simulink model "velocityMode"  (R2022a)
settings: Solver=FixedStepAuto  StartTime=0.0  StopTime=simTime  FixedStep=samplingTime  RelTol=1e-3
values from neighbouring files (symbols this model uses):
  coulombTorqueNegative = theta(4)/theta(2)    [LeastSquare.m]    (also in leastSquare.m; velRide.m = resultFitNeg(2))
  coulombTorquePositive = theta(3)/theta(2)    [LeastSquare.m]    (also in leastSquare.m; velRide.m = resultFitPos(2))
  inertia = 1/K_w    [LeastSquare.m]    (also in leastSquare.m)
  viscousDamping = -inertia*p_w    [LeastSquare.m]    (also in leastSquare.m; velRide.m = (viscousDampingPos+viscousDampingNeg)/2; velocityRide.m = (viscousDampingPos+viscousDampingNeg)/2)
libraries: slpidlib x1
settings Model: Creator=kose  LastModifiedBy=kose
settings DataIOCC: SaveFormat=Array

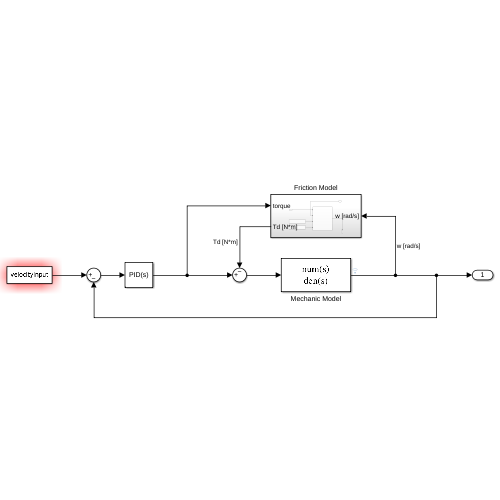
[thumbnail: Simulink's stored preview of the top-level diagram]
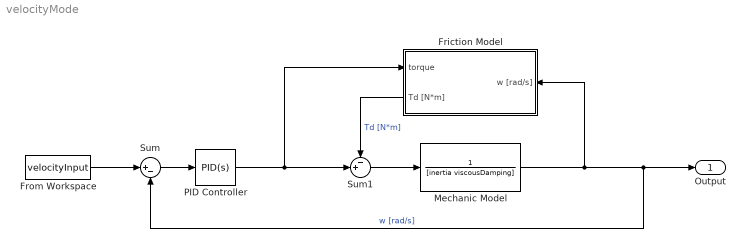
== system velocityMode ==
  Friction Model : Subsystem
      settings: PortSchema="{\"entries\":[{\"content\":{\"sides\":[{\"content\":{\"connectorIds\":[\"In1\"]},\"type\":\"ConnectorPlacement.EquallySpacedRectSide\",\"uuid\":\"8173ecdf-76e4-4809-8dcd-ec0655641a82\"},{\"content\":{\"connectorIds\":[\"In2\",\"Out1\"],\"side\":\"RIGHT\"},\"type\":\"ConnectorPlacement.EquallySpacedRectSide\",\"uuid\":\"02bfb555-c54c-45db-8ee8-f3cb4a7ead24\"},{\"content\":{\"connectorIds\":[],\"side\":\"TOP\"},\"type\":\"ConnectorPlacement.EquallySpacedRectSide\",\"uuid\":\"776da3c7-b053-4a98-8e1b-c60377d5559b\"}]},\"type\":\"ConnectorPlacement.EquallySpacedConnector\",\"uuid\":\"773d656e-d403-490b-8d7a-ce1c081af26d\"}],\"packageUris\":[\"http://schema.mathworks.com/mf0/Connector/R2020b\"],\"version\":\"1.0\"}"
  From Workspace : FromWorkspace  VariableName=velocityInput
  Mechanic Model : TransferFcn  Denominator=[inertia viscousDamping]
  PID Controller : slpidlib/PID Controller  Controller=PID  Form=Parallel  TimeDomain=Continuous-time  UseExternalTs=off  SampleTime=-1  IntegratorMethod=Forward Euler  FilterMethod=Forward Euler  ControllerParametersSource=internal  P=1  I=1  UseKiTs=off  D=0  N=100  UseFilter=on  TunerSelectOption=Transfer Function Based (PID Tuner App)  InitialConditionSource=internal  InitialConditionForIntegrator=0  InitialConditionForFilter=0  DifferentiatorICPrevScaledInput=0  ExternalReset=none  TrackingMode=off  Kt=1  LimitOutput=off  SatLimitsSource=internal  UpperSaturationLimit=inf  LowerSaturationLimit=-inf  LinearizeAsGain=on  AntiWindupMode=none  Kb=1  POutMin=[]  POutMax=[]  IOutMin=[]  IOutMax=[]  DOutMin=[]  DOutMax=[]  NOutMin=[]  NOutMax=[]  SumOutMin=[]  SumOutMax=[]  SaturationOutMin=[]  SaturationOutMax=[]  PParamMin=[]  PParamMax=[]  IParamMin=[]  IParamMax=[]  DParamMin=[]  DParamMax=[]  NParamMin=[]  NParamMax=[]  KbParamMin=[]  KbParamMax=[]  KtParamMin=[]  KtParamMax=[]  KbOutMin=[]  KbOutMax=[]  KtOutMin=[]  KtOutMax=[]  IntegratorOutMin=[]  IntegratorOutMax=[]  FilterOutMin=[]  FilterOutMax=[]  SumI1OutMin=[]  SumI1OutMax=[]  SumI2OutMin=[]  SumI2OutMax=[]  SumI3OutMin=[]  SumI3OutMax=[]  SumI4OutMin=[]  SumI4OutMax=[]  SumDOutMin=[]  SumDOutMax=[]  DifferentiatorOutMin=[]  DifferentiatorOutMax=[]  FilterDiffOutCoefMin=[]  FilterDiffOutCoefMax=[]  ReciprocalOutMin=[]  ReciprocalOutMax=[]  SumDenOutMin=[]  SumDenOutMax=[]  SumNumOutMin=[]  SumNumOutMax=[]  DivideOutMin=[]  DivideOutMax=[]  UdiffTsProdOutMin=[]  UdiffTsProdOutMax=[]  NTsProdOutMin=[]  NTsProdOutMax=[]  UintegralTsProdOutMin=[]  UintegralTsProdOutMax=[]  UngainTsProdOutMin=[]  UngainTsProdOutMax=[]  IntegratorContinuousStateAttributes=''  IntegratorStateMustResolveToSignalObject=off  IntegratorRTWStateStorageClass=Auto  FilterContinuousStateAttributes=''  FilterStateMustResolveToSignalObject=off  FilterRTWStateStorageClass=Auto  ParallelPVariant=InternalParameters  IdealPVariant=Disabled  IVariant=InternalParameters  DVariant=InternalParameters  IntegratorVariant=Continuous  SatVariant=Disabled  AWVariant=Passthrough  PCopyVariant=Disabled  TRVariant=Disabled  FdbkBlocksVariant=Forward  IdealPFdbkVariant=Disabled  SatFdbkVariant=Disabled  DerivativeFilterVariant=ContFilter  NVariant=InternalParameters  NCopyVariant=Disabled  FilterICVariant=InternalICsFilter  IntegratorICVariant=InternalICs  ExternalResetVariant=Disabled  TRSumVariant=Passthrough  SumFdbkVariant=Disabled  SumVariant=Sum_PID  TsampFilterVariant=InternalTs  TsampNgainVariant=Passthrough  TsampIntegralVariant=Passthrough  ExternalSaturationOutDataTypeStr=Inherit: Same as second input  aMode=0
  Sum : Sum  Inputs=|+-
  Sum1 : Sum  Inputs=-+|
  Output : Outport
  wires:
  Mechanic Model/1 -> Friction Model/1(w [rad/s]), Output/1, Sum/2  "w [rad/s]"
  Sum1/1 -> Mechanic Model/1
  Friction Model/1(Td [N*m]) -> Sum1/1  "Td [N*m]"
  PID Controller/1 -> Friction Model/2(torque), Sum1/2
  Sum/1 -> PID Controller/1
  From Workspace/1 -> Sum/1

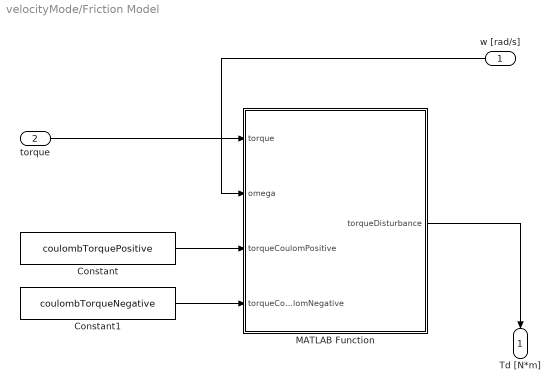
== system velocityMode/Friction Model ==
  w [rad/s] : Inport
  torque : Inport  Port=2
  Constant : Constant  Value=coulombTorquePositive
  Constant1 : Constant  Value=coulombTorqueNegative
  MATLAB Function : MATLAB Function  TreatAsAtomicUnit=on
  Td [N*m] : Outport
  wires:
  w [rad/s]/1 -> MATLAB Function/2(omega)
  Constant/1 -> MATLAB Function/3(torqueCoulomPositive)
  torque/1 -> MATLAB Function/1(torque)
  MATLAB Function/1(torqueDisturbance) -> Td [N*m]/1
  Constant1/1 -> MATLAB Function/4(torqueCoulomNegative)

== matlab function velocityMode/Friction Model/MATLAB Function ==
  data: torque input; torqueDisturbance output; omega input; torqueCoulomPositive input; torqueCoulomNegative input
function torqueDisturbance = fcn(torque, omega, torqueCoulomPositive, torqueCoulomNegative)

if omega > 0
    torqueDisturbance = torqueCoulomPositive;
elseif omega < 0
    torqueDisturbance = torqueCoulomNegative;    
elseif omega == 0 &&  torque < torqueCoulomPositive
    torqueDisturbance = torque;
elseif omega == 0 && torque < torqueCoulomNegative
    torqueDisturbance = torque;
else
    torqueDisturbance = 0;
end
end
